simulink model "conversion_code"  (Simulink 6.1)
settings: Solver=ode45  StartTime=0.0  StopTime=0.1  RelTol=1e-3
libraries: commdigbbndpm2 x2, dspbuff3 x2, commchan2 x1, commrandsrc2 x1, commsink2 x1
settings Model: LastModifiedBy=Administrator

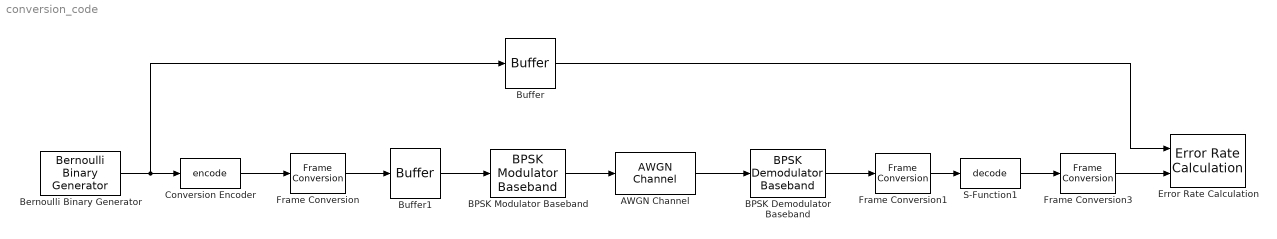
== system conversion_code ==
  AWGN Channel : commchan2/AWGN Channel  seed=67  noiseMode="Signal to noise ratio  (Eb/No)"  EbNodB=SNR  EsNodB=10  SNRdB=10  bitsPerSym=1  Ps=1  Tsym=1e-5  variance=1
  BPSK Demodulator Baseband : commdigbbndpm2/BPSK Demodulator Baseband  Ph=0  numSamp=1
  BPSK Modulator Baseband : commdigbbndpm2/BPSK Modulator Baseband  Ph=0  numSamp=1
  Bernoulli Binary Generator : commrandsrc2/Bernoulli Binary Generator  P=0.5  seed=61  Ts=1e-5  frameBased=off  sampPerFrame=1  orient=off
  Buffer : dspbuff3/Buffer  N=20  V=0  ic=0
  Buffer1 : dspbuff3/Buffer  N=40  V=0  ic=0
  Conversion Encoder : S-Function  FunctionName=encode
  Error Rate Calculation : commsink2/Error Rate Calculation  N=0  st_delay=0  cp_mode=Entire frame  subframe=[]  PMode=Workspace  WsName=BitErrorRate  RsMode2=off  stop=off  numErr=100  maxBits=1e6
  Frame Conversion : FrameConversion
  Frame Conversion1 : FrameConversion  OutFrame=Sample based
  Frame Conversion3 : FrameConversion
  S-Function1 : S-Function  FunctionName=decode
  wires:
  Bernoulli Binary Generator/1 -> Conversion Encoder/1, Buffer/1
  BPSK Modulator Baseband/1 -> AWGN Channel/1
  Conversion Encoder/1 -> Frame Conversion/1
  Frame Conversion/1 -> Buffer1/1
  BPSK Demodulator Baseband/1 -> Frame Conversion1/1
  Frame Conversion1/1 -> S-Function1/1
  S-Function1/1 -> Frame Conversion3/1
  Buffer/1 -> Error Rate Calculation/1
  AWGN Channel/1 -> BPSK Demodulator Baseband/1
  Buffer1/1 -> BPSK Modulator Baseband/1
  Frame Conversion3/1 -> Error Rate Calculation/2
